simulink model "prak1SPK"  (R2015b)
settings: Solver=VariableStepAuto  StartTime=0.0  StopTime=10.0  RelTol=1e-3
libraries: simulink x1
settings Model: Creator=wafiq  LastModifiedBy=wafiq

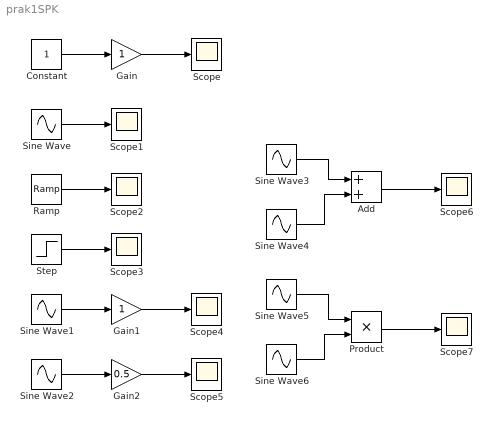
== system prak1SPK ==
  Add : Sum
  Constant : Constant
  Gain : Gain
  Gain1 : Gain
  Gain2 : Gain  Gain=0.5
  Product : Product
  Ramp : simulink/Sources/Ramp  slope=2  start=0  X0=0
  Scope{,1..7} (8 alike) : Scope
  Sine Wave : Sin  Amplitude=2  SampleTime=0
  Sine Wave{1..3,5} (4 alike) : Sin  SampleTime=0
  Sine Wave4 : Sin  Amplitude=2  Frequency=2  SampleTime=0
  Sine Wave6 : Sin  Amplitude=2  Frequency=2  SampleTime=0
  Step : Step  Time=2  SampleTime=0
  wires:
  Constant/1 -> Gain/1
  Gain/1 -> Scope/1
  Ramp/1 -> Scope2/1
  Sine Wave/1 -> Scope1/1
  Step/1 -> Scope3/1
  Sine Wave1/1 -> Gain1/1
  Gain1/1 -> Scope4/1
  Sine Wave2/1 -> Gain2/1
  Gain2/1 -> Scope5/1
  Sine Wave3/1 -> Add/1
  Sine Wave4/1 -> Add/2
  Sine Wave5/1 -> Product/1
  Sine Wave6/1 -> Product/2
  Add/1 -> Scope6/1
  Product/1 -> Scope7/1
